simulink model "chap6_11sim"  (Simulink 6.3)
settings: Solver=ode45  StartTime=0.0  StopTime=10  RelTol=1e-3
settings Model: LastModifiedBy=Administrator  ExtModeTrigMode=oneshot  ExtModeArmWhenConnect=off  StrictBusMsg=None
settings DataIOCC: LimitDataPoints=off  SignalLoggingName=sigsOut
settings OptimizationCC: BooleanDataType=off
settings DebuggingCC: SolverPrmCheckMsg=none
settings HardwareCC: TargetUnknown=on

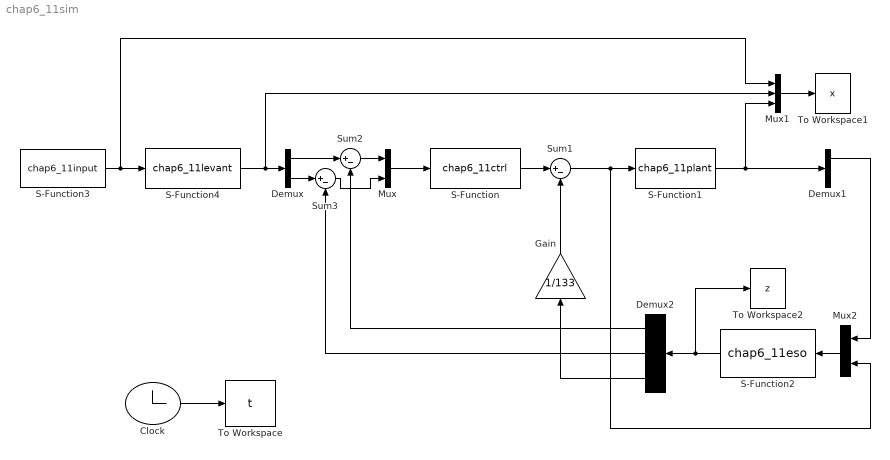
== system chap6_11sim ==
  Clock : Clock
  Demux : Demux  Outputs=2
  Demux1 : Demux  Outputs=3
  Demux2 : Demux  Orientation=left  Outputs=3
  Gain : Gain  Orientation=up  Gain=1/133
  Mux : Mux  Inputs=2
  Mux1 : Mux  Inputs=3
  Mux2 : Mux  Orientation=left  Inputs=2
  S-Function : S-Function  FunctionName=chap6_11ctrl
  S-Function1 : S-Function  FunctionName=chap6_11plant
  S-Function2 : S-Function  Orientation=left  FunctionName=chap6_11eso
  S-Function3 : S-Function  FunctionName=chap6_11input
  S-Function4 : S-Function  FunctionName=chap6_11levant
  Sum1 : Sum  Inputs=|+-  SaturateOnIntegerOverflow=on
  Sum2 : Sum  Inputs=|+-  SaturateOnIntegerOverflow=on
  Sum3 : Sum  Inputs=|+-  SaturateOnIntegerOverflow=on
  To Workspace : ToWorkspace  VariableName=t  SampleTime=-1  SaveFormat=Array
  To Workspace1 : ToWorkspace  VariableName=x  SampleTime=-1  SaveFormat=Array
  To Workspace2 : ToWorkspace  VariableName=z  SampleTime=-1  SaveFormat=Array
  wires:
  Clock/1 -> To Workspace/1
  S-Function1/1 -> Demux1/1, Mux1/3
  S-Function2/1 -> Demux2/1, To Workspace2/1
  Demux2/2 -> Sum3/2
  Demux2/3 -> Gain/1
  Sum1/1 -> S-Function1/1, Mux2/2
  S-Function/1 -> Sum1/1
  Gain/1 -> Sum1/2
  Mux2/1 -> S-Function2/1
  Demux1/1 -> Mux2/1
  S-Function4/1 -> Demux/1, Mux1/2
  Mux/1 -> S-Function/1
  Demux2/1 -> Sum2/2
  Demux/1 -> Sum2/1
  Demux/2 -> Sum3/1
  Sum2/1 -> Mux/1
  Sum3/1 -> Mux/2
  Mux1/1 -> To Workspace1/1
  S-Function3/1 -> S-Function4/1, Mux1/1
